simulink model "Day6_Scenario_2"  (R2024a)
settings: Solver=VariableStepAuto  StartTime=0.0  StopTime=10.0  RelTol=1e-3
undefined symbols (not defined in the file): Waypoints
libraries: CarMaker4SL x14
settings Model: Creator=User  LastModifiedBy=User

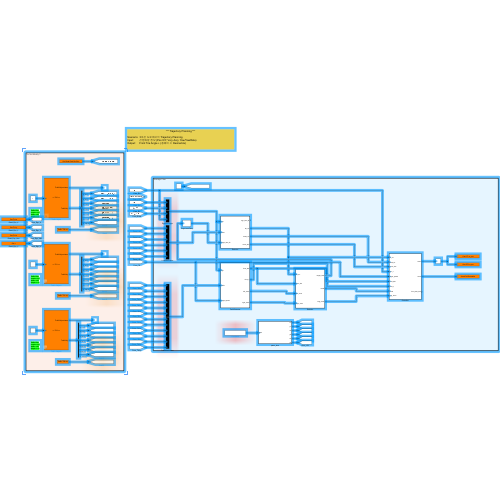
[thumbnail: Simulink's stored preview of the top-level diagram]
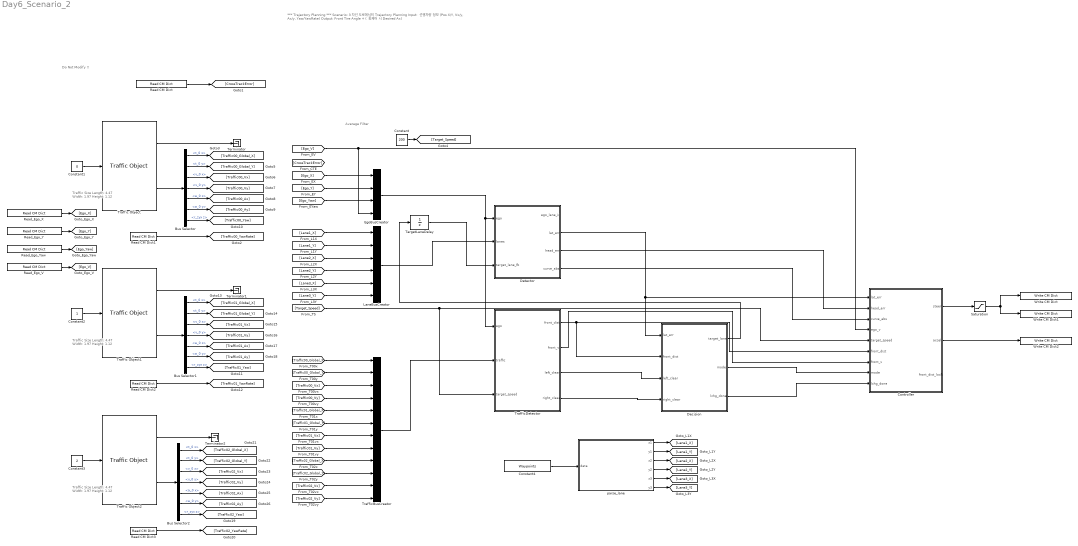
== system Day6_Scenario_2 ==
  note: Traffic Size
      | Length: 4.47
      | Width: 1.97
      | Height: 1.12
  note: *** Trajectory Planning ***
      |
      | Scenario: 3차선 도로에서의 Trajectory Planning
      | Input: 선행차량 정보 (Pos X/Y, Vx/y, Ax/y, Yaw/YawRate)
      | Output: Front Tire Angle + (종제어 시 Desired Ax)
  note: Average Filter
  note: Traffic Size
      | Length: 4.47
      | Width: 1.97
      | Height: 1.12
  note: Traffic Size
      | Length: 4.47
      | Width: 1.97
      | Height: 1.12
  note: Do Not Modify !!
  Bus Selector : BusSelector  OutputSignals=t_0 x,t_0 y,v_0 x,v_0 y,a_0 x,a_0 y,r_zyx z
  Bus Selector1 : BusSelector  OutputSignals=t_0 x,t_0 y,v_0 x,v_0 y,a_0 x,a_0 y,r_zyx z
  Bus Selector2 : BusSelector  OutputSignals=t_0 x,t_0 y,v_0 x,v_0 y,a_0 x,a_0 y,r_zyx z
  Constant : Constant  Value=200
  Constant1 : Constant  Value=0
  Constant2 : Constant
  Constant3 : Constant  Value=2
  Constant4 : Constant  Value=Waypoints
  Controller : MATLAB Function  TreatAsAtomicUnit=on
  Decision : MATLAB Function  TreatAsAtomicUnit=on
  Detector : MATLAB Function  TreatAsAtomicUnit=on
  EgoBusCreator : BusCreator  Inputs=4  OutDataTypeStr=Bus: EgoBus  NonVirtualBus=on
  LaneBusCreator : BusCreator  Inputs=6  OutDataTypeStr=Bus: LaneBus  NonVirtualBus=on
  Read CM Dict : CarMaker4SL/Read CM Dict  xname=Car.Road.Path.DevDist  xsync=off  xstime=Inherited
  Read CM Dict1 : CarMaker4SL/Read CM Dict  xname=Traffic.T00.rzv  xsync=off  xstime=Inherited
  Read CM Dict2 : CarMaker4SL/Read CM Dict  xname=Traffic.T01.rzv  xsync=off  xstime=Inherited
  Read CM Dict3 : CarMaker4SL/Read CM Dict  xname=Traffic.T02.rzv  xsync=off  xstime=Inherited
  Read_Ego_V : CarMaker4SL/Read CM Dict  xname=Car.v  xsync=off  xstime=Continuous
  Read_Ego_X : CarMaker4SL/Read CM Dict  xname=Car.Fr1.tx  xsync=off  xstime=Continuous
  Read_Ego_Y : CarMaker4SL/Read CM Dict  xname=Car.Fr1.ty  xsync=off  xstime=Continuous
  Read_Ego_Yaw : CarMaker4SL/Read CM Dict  xname=Car.Fr1.rz  xsync=off  xstime=Continuous
  Saturation : Saturate  UpperLimit=2  LowerLimit=-2
  TargetLaneDelay : UnitDelay  InitialCondition=int32(1)  SampleTime=-1  HasFrameUpgradeWarning=on
  Terminator : Terminator
  Terminator1 : Terminator
  Terminator2 : Terminator
  Traffic Object : CarMaker4SL/Traffic Object  xname=T00  ximode=Traffic Id  xstime=Inherited
      settings: SourceProductName=CarMaker4SL
  Traffic Object1 : CarMaker4SL/Traffic Object  xname=T01  ximode=Traffic Id  xstime=Inherited
      settings: SourceProductName=CarMaker4SL
  Traffic Object2 : CarMaker4SL/Traffic Object  xname=T02  ximode=Traffic Id  xstime=Inherited
      settings: SourceProductName=CarMaker4SL
  TrafficBusCreator : BusCreator  Inputs=12  OutDataTypeStr=Bus: TrafficBus  NonVirtualBus=on
  TrafficDetector : MATLAB Function  TreatAsAtomicUnit=on
  Write CM Dict : CarMaker4SL/Write CM Dict  xname=Car.CFL.rz_ext  xsync=off
  Write CM Dict1 : CarMaker4SL/Write CM Dict  xname=Car.CFR.rz_ext  xsync=off
  Write CM Dict2 : CarMaker4SL/Write CM Dict  xname=AccelCtrl.DesiredAx  xsync=off
  parse_lane : MATLAB Function  TreatAsAtomicUnit=on
  wires:
  Traffic Object2/2 -> Bus Selector2/1
  Read CM Dict/1 -> [CrossTrackError]
  [Traffic00_Global_X] -> TrafficBusCreator/1
  [Traffic01_Vx] -> TrafficBusCreator/7
  parse_lane/2(y1) -> [Lane1_Y]
  Bus Selector/6 -> [Traffic00_Ay]  "<a_0 y>"
  [Traffic02_Global_X] -> TrafficBusCreator/9
  Traffic Object1/2 -> Bus Selector1/1
  [Ego_Y] -> EgoBusCreator/2
  [Traffic01_Global_X] -> TrafficBusCreator/5
  Constant4/1 -> parse_lane/1(data)
  Decision/2(mode) -> Controller/8(mode)
  Read_Ego_V/1 -> [Ego_V]
  Traffic Object/1 -> Terminator/1
  [Traffic01_Vy] -> TrafficBusCreator/8
  [Traffic00_Vy] -> TrafficBusCreator/4
  TrafficDetector/3(left_clear) -> Decision/3(left_clear)
  parse_lane/6(y3) -> [Lane3_Y]
  Decision/1(target_lane) -> TargetLaneDelay/1
  [Traffic00_Global_Y] -> TrafficBusCreator/2
  parse_lane/1(x1) -> [Lane1_X]
  TrafficDetector/2(front_v) -> Controller/7(front_v)
  [Traffic02_Vx] -> TrafficBusCreator/11
  Bus Selector/1 -> [Traffic00_Global_X]  "<t_0 x>"
  Bus Selector2/1 -> [Traffic02_Global_X]  "<t_0 x>"
  Detector/2(lat_err) -> Decision/1(lat_err), Controller/1(lat_err)
  Detector/4(curve_abs) -> Controller/3(curve_abs)
  Constant3/1 -> Traffic Object2/1
  TrafficBusCreator/1 -> TrafficDetector/2(traffic)
  [Traffic02_Global_Y] -> TrafficBusCreator/10
  Bus Selector2/5 -> [Traffic02_Ax]  "<a_0 x>"
  TrafficDetector/4(right_clear) -> Decision/4(right_clear)
  Detector/3(head_err) -> Controller/2(head_err)
  parse_lane/5(x3) -> [Lane3_X]
  [Ego_Yaw] -> EgoBusCreator/3
  Constant1/1 -> Traffic Object/1
  Traffic Object2/1 -> Terminator2/1
  LaneBusCreator/1 -> Detector/2(lanes)
  [Traffic00_Vx] -> TrafficBusCreator/3
  [Lane2_X] -> LaneBusCreator/3
  TargetLaneDelay/1 -> Detector/3(target_lane_fb)
  Traffic Object1/1 -> Terminator1/1
  Bus Selector2/3 -> [Traffic02_Vx]  "<v_0 x>"
  [Lane1_X] -> LaneBusCreator/1
  [Lane3_Y] -> LaneBusCreator/6
  [Lane3_X] -> LaneBusCreator/5
  Bus Selector2/7 -> [Traffic02_Yaw]  "<r_zyx z>"
  Read CM Dict2/1 -> [Traffic01_YawRate]
  Constant2/1 -> Traffic Object1/1
  [Ego_V] -> Controller/4(ego_v), EgoBusCreator/4
  EgoBusCreator/1 -> TrafficDetector/1(ego), Detector/1(ego)
  Bus Selector1/7 -> [Traffic01_Yaw]  "<r_zyx z>"
  [Traffic02_Vy] -> TrafficBusCreator/12
  Bus Selector1/4 -> [Traffic01_Vy]  "<v_0 y>"
  Read_Ego_Y/1 -> [Ego_Y]
  Decision/3(lchg_done) -> Controller/9(lchg_done)
  Bus Selector/7 -> [Traffic00_Yaw]  "<r_zyx z>"
  parse_lane/3(x2) -> [Lane2_X]
  parse_lane/4(y2) -> [Lane2_Y]
  Bus Selector1/6 -> [Traffic01_Ay]  "<a_0 y>"
  TrafficDetector/1(front_dist) -> Controller/6(front_dist), Decision/2(front_dist)
  [Lane1_Y] -> LaneBusCreator/2
  Bus Selector1/3 -> [Traffic01_Vx]  "<v_0 x>"
  Bus Selector1/5 -> [Traffic01_Ax]  "<a_0 x>"
  Bus Selector1/2 -> [Traffic01_Global_Y]  "<t_0 y>"
  Read CM Dict3/1 -> [Traffic02_YawRate]
  Bus Selector/2 -> [Traffic00_Global_Y]  "<t_0 y>"
  Read_Ego_X/1 -> [Ego_X]
  [Traffic01_Global_Y] -> TrafficBusCreator/6
  Read CM Dict1/1 -> [Traffic00_YawRate]
  Controller/2(accel) -> Write CM Dict2/1
  [Lane2_Y] -> LaneBusCreator/4
  Read_Ego_Yaw/1 -> [Ego_Yaw]
  Constant/1 -> [Target_Speed]
  Traffic Object/2 -> Bus Selector/1
  Saturation/1 -> Write CM Dict1/1, Write CM Dict/1
  Bus Selector/4 -> [Traffic00_Vy]  "<v_0 y>"
  [Ego_X] -> EgoBusCreator/1
  Bus Selector1/1 -> [Traffic01_Global_X]  "<t_0 x>"
  Bus Selector/5 -> [Traffic00_Ax]  "<a_0 x>"
  Controller/1(steer) -> Saturation/1
  Bus Selector2/4 -> [Traffic02_Vy]  "<v_0 y>"
  [Target_Speed] -> TrafficDetector/3(target_speed), Controller/5(target_speed)
  Bus Selector2/6 -> [Traffic02_Ay]  "<a_0 y>"
  Bus Selector/3 -> [Traffic00_Vx]  "<v_0 x>"
  Bus Selector2/2 -> [Traffic02_Global_Y]  "<t_0 y>"

== matlab function Day6_Scenario_2/TrafficDetector ==
  data: ego input Bus: EgoBus size=[1 1]; front_dist output double size=[1 1]; traffic input Bus: TrafficBus size=[1 1]; target_speed input double size=[1 1]; front_v output double size=[1 1]; left_clear output boolean size=[1 1]; right_clear output boolean size=[1 1]
function [front_dist, front_v, left_clear, right_clear] = traffic_detector(ego, traffic, target_speed)
%#codegen
    % --- 버스 필드 unpack ---
    ego_x = ego.x; ego_y = ego.y; ego_yaw = ego.yaw;
    t00_x = traffic.t00_x; t00_y = traffic.t00_y; t00_vx = traffic.t00_vx; t00_vy = traffic.t00_vy;
    t01_x = traffic.t01_x; t01_y = traffic.t01_y; t01_vx = traffic.t01_vx; t01_vy = traffic.t01_vy;
    t02_x = traffic.t02_x; t02_y = traffic.t02_y; t02_vx = traffic.t02_vx; t02_vy = traffic.t02_vy;
    
    LOOK_FRONT = 30.0;  LANE_HALF_W = 2.0;
    cy = cos(ego_yaw); sy = sin(ego_yaw);
    dxg = t00_x - ego_x; dyg = t00_y - ego_y;
    t00_xL =  cy*dxg + sy*dyg;  t00_yL = -sy*dxg + cy*dyg;
    dxg = t01_x - ego_x; dyg = t01_y - ego_y;
    t01_xL =  cy*dxg + sy*dyg;  t01_yL = -sy*dxg + cy*dyg;
    dxg = t02_x - ego_x; dyg = t02_y - ego_y;
    t02_xL =  cy*dxg + sy*dyg;  t02_yL = -sy*dxg + cy*dyg;
    front_dist = 1e9;  front_v = target_speed;
    if t00_xL > 0 && t00_xL < LOOK_FRONT && abs(t00_yL) < LANE_HALF_W
        if t00_xL < front_dist, front_dist = t00_xL; front_v = sqrt(t00_vx^2 + t00_vy^2); end
    end
    if t01_xL > 0 && t01_xL < LOOK_FRONT && abs(t01_yL) < LANE_HALF_W
        if t01_xL < front_dist, front_dist = t01_xL; front_v = sqrt(t01_vx^2 + t01_vy^2); end
    end
    if t02_xL > 0 && t02_xL < LOOK_FRONT && abs(t02_yL) < LANE_HALF_W
        if t02_xL < front_dist, front_dist = t02_xL; front_v = sqrt(t02_vx^2 + t02_vy^2); end
    end
    left_clear = true;  right_clear = true;
    if t00_xL > -5 && t00_xL < 20 && t00_yL >  LANE_HALF_W && t00_yL <  3*LANE_HALF_W, left_clear = false; end
    if t01_xL > -5 && t01_xL < 20 && t01_yL >  LANE_HALF_W && t01_yL <  3*LANE_HALF_W, left_clear = false; end
    if t02_xL > -5 && t02_xL < 20 && t02_yL >  LANE_HALF_W && t02_yL <  3*LANE_HALF_W, left_clear = false; end
    if t00_xL > -5 && t00_xL < 20 && t00_yL < -LANE_HALF_W && t00_yL > -3*LANE_HALF_W, right_clear = false; end
    if t01_xL > -5 && t01_xL < 20 && t01_yL < -LANE_HALF_W && t01_yL > -3*LANE_HALF_W, right_clear = false; end
    if t02_xL > -5 && t02_xL < 20 && t02_yL < -LANE_HALF_W && t02_yL > -3*LANE_HALF_W, right_clear = false; end
end

== matlab function Day6_Scenario_2/Detector ==
  data: ego input Bus: EgoBus size=[1 1]; ego_lane_id output int32 size=[1 1]; lanes input Bus: LaneBus size=[1 1]; target_lane_fb input int32 size=[1 1]; lat_err output double size=[1 1]; head_err output double size=[1 1]; curve_abs output double size=[1 1]
function [ego_lane_id, lat_err, head_err, curve_abs] = detector(ego, lanes, target_lane_fb)
%#codegen
    % --- 버스 필드 unpack ---
    ego_x = ego.x; ego_y = ego.y; ego_yaw = ego.yaw;
    x1 = lanes.x1; y1 = lanes.y1;
    x2 = lanes.x2; y2 = lanes.y2;
    x3 = lanes.x3; y3 = lanes.y3;
    
    % ego 현재 가장 가까운 lane
    d1 = nearest_d2(x1, y1, ego_x, ego_y);
    d2 = nearest_d2(x2, y2, ego_x, ego_y);
    d3 = nearest_d2(x3, y3, ego_x, ego_y);
    if d1 <= d2 && d1 <= d3
        ego_lane_id = int32(1);
    elseif d2 <= d3
        ego_lane_id = int32(2);
    else
        ego_lane_id = int32(3);
    end
    
    % target_lane_fb 기준 오차 + 곡률
    if target_lane_fb == int32(1)
        [lat_err, head_err, curve_abs] = process_lane(x1, y1, ego_x, ego_y, ego_yaw);
    elseif target_lane_fb == int32(2)
        [lat_err, head_err, curve_abs] = process_lane(x2, y2, ego_x, ego_y, ego_yaw);
    else
        [lat_err, head_err, curve_abs] = process_lane(x3, y3, ego_x, ego_y, ego_yaw);
    end
end

function d2 = nearest_d2(xa, ya, ex, ey)
    d2 = 1e12;
    N = int32(numel(xa));
    for i = 1:N
        dxk = xa(i) - ex; dyk = ya(i) - ey;
        v = dxk*dxk + dyk*dyk;
        if v < d2, d2 = v; end
    end
end

function [lat_err, head_err, curve_abs] = process_lane(xa, ya, ex, ey, eyaw)
    N = int32(numel(xa));
    best_i = int32(1);  best_d2 = 1e12;
    for i = 1:N
        dxk = xa(i) - ex; dyk = ya(i) - ey;
        v = dxk*dxk + dyk*dyk;
        if v < best_d2, best_d2 = v; best_i = i; end
    end
    look_i = best_i + int32(5);
    if look_i > N, look_i = N; end
    if look_i > best_i
        path_yaw = atan2(ya(look_i)-ya(best_i), xa(look_i)-xa(best_i));
    elseif best_i > int32(1)
        path_yaw = atan2(ya(best_i)-ya(best_i-1), xa(best_i)-xa(best_i-1));
    else
        path_yaw = eyaw;
    end
    dxr = ex - xa(best_i);  dyr = ey - ya(best_i);
    lat_err = -sin(path_yaw)*dxr + cos(path_yaw)*dyr;
    head_err = path_yaw - eyaw;
    while head_err >  pi, head_err = head_err - 2*pi; end
    while head_err < -pi, head_err = head_err + 2*pi; end
    curve_abs = 0;
    i1 = best_i + int32(3); i2 = best_i + int32(10); i3 = best_i + int32(17);
    if i1 > N, i1 = N; end
    if i2 > N, i2 = N; end
    if i3 > N, i3 = N; end
    if i1 < i2 && i2 < i3
        yaw1 = atan2(ya(i2)-ya(i1), xa(i2)-xa(i1));
        yaw2 = atan2(ya(i3)-ya(i2), xa(i3)-xa(i2));
        dyaw = yaw2 - yaw1;
        while dyaw >  pi, dyaw = dyaw - 2*pi; end
        while dyaw < -pi, dyaw = dyaw + 2*pi; end
        ds = sqrt((xa(i3)-xa(i1))^2 + (ya(i3)-ya(i1))^2);
        if ds > 0.1, curve_abs = abs(dyaw)/ds; end
    end
end

== matlab function Day6_Scenario_2/Decision ==
  data: lat_err input double size=[1 1]; target_lane output int32 size=[1 1]; front_dist input double size=[1 1]; left_clear input boolean size=[1 1]; right_clear input boolean size=[1 1]; mode output int32 size=[1 1]; lchg_done output boolean size=[1 1]
function [target_lane, mode, lchg_done] = decision(lat_err, front_dist, left_clear, right_clear)
%#codegen
    LCHG_TRIG_D = 25.0;
    LAT_ARRIVED = 0.5;
    MODE_ACC = int32(0);
    MODE_LCHG = int32(1);
    
    persistent target_lane_p mode_p lchg_done_p did_init
    if isempty(did_init)
        target_lane_p = int32(1);
        mode_p = MODE_ACC;
        lchg_done_p = false;
        did_init = true;
    end
    
    % --- 출력은 현재 state (이번 step 입력 의존 X → 루프 차단) ---
    target_lane = target_lane_p;
    mode        = mode_p;
    lchg_done   = lchg_done_p;
    
    % --- 다음 step 용 state 갱신 ---
    if mode_p == MODE_ACC
        if front_dist < LCHG_TRIG_D
            if left_clear && target_lane_p < int32(3)
                target_lane_p = target_lane_p + int32(1);
                mode_p = MODE_LCHG;
                lchg_done_p = true;
            elseif right_clear && target_lane_p > int32(1)
                target_lane_p = target_lane_p - int32(1);
                mode_p = MODE_LCHG;
                lchg_done_p = true;
            end
        end
    else
        if abs(lat_err) < LAT_ARRIVED
            mode_p = MODE_ACC;
        end
    end
end

== matlab function Day6_Scenario_2/Controller ==
  data: lat_err input double size=[1 1]; steer output double size=[1 1]; head_err input double size=[1 1]; curve_abs input double size=[1 1]; ego_v input double size=[1 1]; target_speed input double size=[1 1]; front_dist input double size=[1 1]; front_v input double size=[1 1]; mode input int32 size=[1 1]; lchg_done input boolean size=[1 1]; accel output double size=[1 1]; front_dist_lock output double size=[1 1]
function [steer, accel, front_dist_lock] = controller(...
    lat_err, head_err, curve_abs, ego_v, target_speed, ...
    front_dist, front_v, mode, lchg_done)
%#codegen
    STEER_LIM = 0.5;
    ACCEL_LIM = 4.0;
    K_STANLEY = 0.5;
    KP_HEAD   = 1.0;
    KP_SPD    = 1.0;
    MAX_SPEED = 25;
    LOOK_FRONT = 30.0;
    CURVE_TH          = 0.008;
    SHARP_CURVE_TH    = 0.018;
    CURVE_SPEED       = 10.0;
    SHARP_CURVE_SPEED = 7.5;
    MODE_LCHG = int32(1);
    
    ts = target_speed;
    if ts > 20, ts = ts / 3.6; end
    if ts > MAX_SPEED, ts = MAX_SPEED; end
    if ts < 0, ts = 0; end
    
    % --- Stanley 조향 ---
    v_safe = ego_v;
    if v_safe < 1, v_safe = 1; end
    steer = KP_HEAD * head_err - atan2(K_STANLEY * lat_err, v_safe);
    if steer >  STEER_LIM, steer =  STEER_LIM; end
    if steer < -STEER_LIM, steer = -STEER_LIM; end
    
    % --- 종방향 ACC + 코너 감속 ---
    desired_v = ts;
    if curve_abs > SHARP_CURVE_TH
        if desired_v > SHARP_CURVE_SPEED, desired_v = SHARP_CURVE_SPEED; end
    elseif curve_abs > CURVE_TH
        if desired_v > CURVE_SPEED, desired_v = CURVE_SPEED; end
    end
    if front_dist < LOOK_FRONT
        time_gap = 1.5;
        safe_v = front_v + (front_dist - time_gap*ego_v) * 0.3;
        if safe_v < desired_v, desired_v = safe_v; end
    end
    if desired_v < 0, desired_v = 0; end
    
    spd_err = desired_v - ego_v;
    if spd_err < -3
        accel = 2.0 * spd_err;
    else
        accel = KP_SPD * spd_err;
    end
    if accel >  ACCEL_LIM, accel =  ACCEL_LIM; end
    if accel < -ACCEL_LIM, accel = -ACCEL_LIM; end
    
    % --- Switch lock (front_dist_lock 출력) ---
    if mode == MODE_LCHG || lchg_done
        front_dist_lock = 0;
    else
        front_dist_lock = front_dist;
    end
end

== matlab function Day6_Scenario_2/parse_lane ==
  data: data input double size=[654 4]; x1 output double size=[207 1]; y1 output double size=[207 1]; x2 output double size=[222 1]; y2 output double size=[222 1]; x3 output double size=[225 1]; y3 output double size=[225 1]
function [x1,y1,x2,y2,x3,y3] = parse_lane(data)
%#codegen
    % fixed-size 출력 — build_day6_planning 이 자동 갱신
    N1 = 207;
    N2 = 222;
    N3 = 225;
    x1 = zeros(N1, 1);
    y1 = zeros(N1, 1);
    x2 = zeros(N2, 1);
    y2 = zeros(N2, 1);
    x3 = zeros(N3, 1);
    y3 = zeros(N3, 1);
    i1 = int32(0);
    i2 = int32(0);
    i3 = int32(0);
    N  = int32(size(data, 1));
    for k = 1:N
        lk = data(k, 4);
        xk = data(k, 2);
        yk = data(k, 3);
        if lk == 1
            if i1 < int32(N1)
                i1 = i1 + int32(1);
                x1(i1) = xk;
                y1(i1) = yk;
            end
        elseif lk == 2
            if i2 < int32(N2)
                i2 = i2 + int32(1);
                x2(i2) = xk;
                y2(i2) = yk;
            end
        elseif lk == 3
            if i3 < int32(N3)
                i3 = i3 + int32(1);
                x3(i3) = xk;
                y3(i3) = yk;
            end
        end
    end
end
